simulink model "model_estado"  (R2022b)
settings: Solver=ode45  StartTime=0.0  StopTime=0.06  RelTol=1e-3  EnableMultiTasking=on
values from neighbouring files (symbols this model uses):
  Bm = 1e-04    (= 0.0001)    [loop_estado.m]    (also in loop_pid.m = 5e-08; var_estado.m; var_pid.m = 5e-08)
  J = 1e-04    (= 0.0001)    [loop_estado.m]    (also in loop_pid.m = 8e-08; var_estado.m; var_pid.m = 8e-08)
  ka = 0.16    [loop_estado.m]    (also in loop_pid.m = 0.2; var_estado.m; var_pid.m = 0.2)
  La = 0.0066    [loop_estado.m]    (also in loop_pid.m = 0.002; var_estado.m; var_pid.m = 0.002)
  ra = 3.15    [loop_estado.m]    (also in loop_pid.m = 200; var_estado.m; var_pid.m = 200)
  u_lim = 30    [loop_estado.m]    (also in sim_estado.m = ULIM(i); sim_pid.m = ULIM(i); var_estado.m)
undefined symbols (not defined in the file or in its folder): KF
settings Model: Creator=12549703  LastModifiedBy=andre
settings SolverCC: AlgebraicLoopSolver=TrustRegion
settings DataIOCC: LimitDataPoints=on  SaveFormat=Array  ReturnWorkspaceOutputs=off
settings OptimizationCC: LifeSpan=inf
settings DebuggingCC: UnconnectedInputMsg=warning  UnconnectedOutputMsg=warning  UnconnectedLineMsg=warning  SFUnexpectedBacktrackingDiag=warning  SFNoUnconditionalDefaultTransitionDiag=warning  SFExecutionAtInitializationDiag=none  SFMachineParentedDataDiag=warning  ArithmeticOperatorsInVariantConditions=warning
settings HardwareCC: ProdBitPerPointer=32  ProdBitPerSizeT=32  ProdBitPerPtrDiffT=32  ProdLargestAtomicFloat=None  ProdIntDivRoundTo=Undefined  ProdEndianess=Unspecified  ProdWordSize=32  ProdHWDeviceType=32-bit Generic
settings ModelReferenceCC: PropagateSignalLabelsOutOfModel=off
settings SFSimCC: SimUseLocalCustomCode=off  CustomCodeUndefinedFunction=UseInterfaceOnly
settings RTWCC: RTWUseLocalCustomCode=off
settings CodeAppCC: StateflowObjectComments=on
settings GRTTargetCC: TargetLangStandard=C89/C90 (ANSI)
settings ConfigComp: CovMetricSettings=dw  CovSaveCumulativeToWorkspaceVar=on  CovSaveSingleToWorkspaceVar=on  CovExternalEMLEnable=off

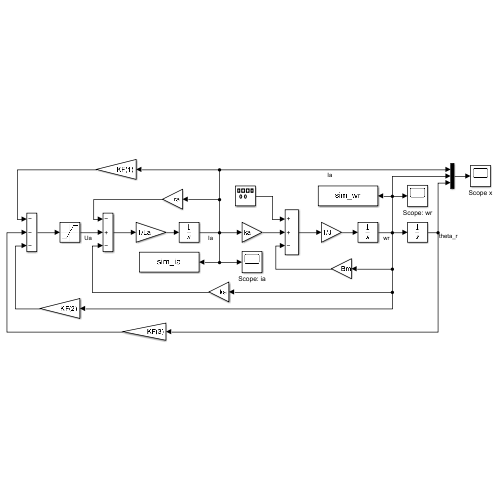
[thumbnail: Simulink's stored preview of the top-level diagram]
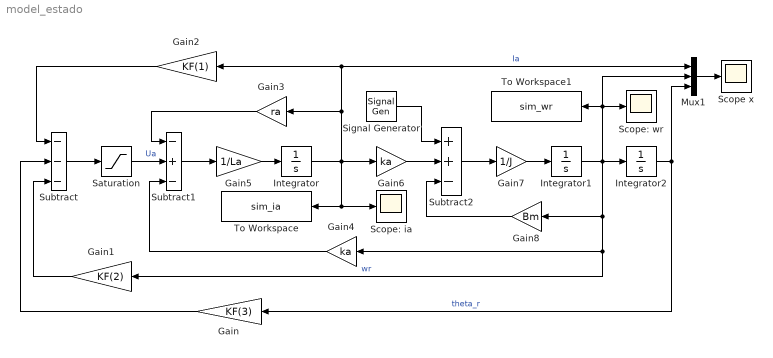
== system model_estado ==
  Gain : Gain  Gain=KF(3)
  Gain1 : Gain  Gain=KF(2)
  Gain2 : Gain  Gain=KF(1)
  Gain3 : Gain  Gain=ra
  Gain4 : Gain  Gain=ka
  Gain5 : Gain  Gain=1/La
  Gain6 : Gain  Gain=ka
  Gain7 : Gain  Gain=1/J
  Gain8 : Gain  Gain=Bm
  Integrator : Integrator  InitialCondition=10
  Integrator1 : Integrator  InitialCondition=25
  Integrator2 : Integrator  InitialCondition=1
  Mux1 : Mux  Inputs=3
  Saturation : Saturate  UpperLimit=u_lim  LowerLimit=-u_lim
  Scope x : Scope
  Scope: ia : Scope
  Scope: wr : Scope
  Signal Generator : SignalGenerator  Units=rad/sec
  Subtract : Sum  Inputs=---
  Subtract1 : Sum  Inputs=-+-
  Subtract2 : Sum  Inputs=++-
  To Workspace : ToWorkspace  VariableName=sim_ia  SaveFormat=Timeseries  SampleTime=-1
  To Workspace1 : ToWorkspace  VariableName=sim_wr  SaveFormat=Timeseries  SampleTime=-1
  wires:
  Gain4/1 -> Subtract1/3
  Gain3/1 -> Subtract1/1
  Subtract1/1 -> Gain5/1
  Gain5/1 -> Integrator/1
  Integrator/1 -> To Workspace/1, Scope: ia/1, Gain2/1, Mux1/1, Gain3/1, Gain6/1  "Ia"
  Gain2/1 -> Subtract/1
  Gain6/1 -> Subtract2/2
  Gain8/1 -> Subtract2/3
  Subtract2/1 -> Gain7/1
  Gain7/1 -> Integrator1/1
  Integrator1/1 -> Integrator2/1, Gain1/1, Gain4/1, Gain8/1, Mux1/2, To Workspace1/1, Scope: wr/1  "wr"
  Integrator2/1 -> Gain/1, Mux1/3  "theta_r"
  Gain1/1 -> Subtract/3
  Gain/1 -> Subtract/2
  Mux1/1 -> Scope x/1
  Subtract/1 -> Saturation/1
  Saturation/1 -> Subtract1/2  "Ua"
  Signal Generator/1 -> Subtract2/1
